simulink model "example8_4"  (R2016b)
settings: Solver=FixedStepDiscrete  StartTime=0.0  StopTime=10.0  RelTol=1e-3  EnableMultiTasking=on
libraries: dspsrcs4 x2, dsparch4 x1, dspadpt3 x1
settings Model: Creator=The MathWorks, Inc.  LastModifiedBy=zhangjin
settings DataIOCC: LimitDataPoints=on  SaveFormat=Array  SignalLoggingName=logsOut
settings OptimizationCC: ExpressionDepthLimit=2147483647  InitFltsAndDblsToZero=on  EfficientMapNaN2IntZero=off  LifeSpan=inf
settings DebuggingCC: SaveWithParameterizedLinksMsg=none  UnderspecifiedInitializationDetection=Classic  MergeDetectMultiDrivingBlocksExec=none  CheckExecutionContextPreStartOutputMsg=on  CheckExecutionContextRuntimeOutputMsg=on  SolverPrmCheckMsg=warning  MultiTaskDSMMsg=warning  MultiTaskCondExecSysMsg=none  FcnCallInpInsideContextMsg=warning  StateNameClashWarn=warning  StrictBusMsg=None  SFUnexpectedBacktrackingDiag=warning  SFNoUnconditionalDefaultTransitionDiag=warning  SFExecutionAtInitializationDiag=none
settings HardwareCC: ProdBitPerPointer=32  ProdBitPerSizeT=32  ProdBitPerPtrDiffT=32  ProdLargestAtomicFloat=None  ProdIntDivRoundTo=Undefined  ProdEndianess=Unspecified  ProdWordSize=32  ProdHWDeviceType=32-bit Generic
settings ModelReferenceCC: UpdateModelReferenceTargets=IfOutOfDate  PropagateSignalLabelsOutOfModel=off
settings GRTTargetCC: TargetFcnLib=ansi_tfl_tmw.mat  TargetLangStandard=C89/C90 (ANSI)  GeneratePreprocessorConditionals=Disable all  CombineOutputUpdateFcns=off  GRTInterface=on
settings ConfigComp: CovMetricSettings=dw  CovHtmlReporting=on  CovSaveCumulativeToWorkspaceVar=on  CovSaveSingleToWorkspaceVar=on  CovExternalEMLEnable=off

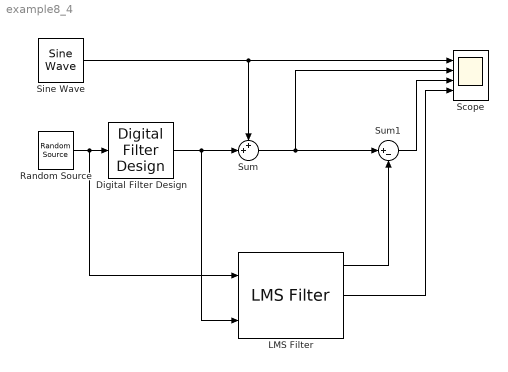
== system example8_4 ==
  Digital Filter Design : dsparch4/Digital Filter Design  mwdsp_browser_bugfix_var=off
  LMS Filter : dspadpt3/LMS Filter  Algo=Normalized LMS  L=32  stepflag=Dialog  mu=0.1  leakage=1.0  ic=0  Adapt=off  resetflag=None  weights=on  secondCoeffMode=User-defined  secondCoeffWordLength=2  secondCoeffFracLength=15  accum2Mode=User-defined  accum2FracLength=20  prodOutput2Mode=User-defined  prodOutput2FracLength=20  prodOutput3Mode=User-defined  prodOutput3FracLength=20  prodOutput4Mode=User-defined  prodOutput4FracLength=20  quotientMode=User-defined  quotientFracLength=20  roundingMode=Floor  overflowMode=off  addnparflag=off
  Random Source : dspsrcs4/Random Source  SrcType=Gaussian  NormMethod=Ziggurat  CltLength=12  MinVal=0  MaxVal=1  MeanVal=0  VarVal=1  RepMode=Specify seed  rawSeed=[23341]  IsInherit=off  SampMode=Discrete  SampTime=0.05  SampFrame=1  DataType=Double  OutComplex=Real  OutputFrames=on
  Scope : Scope  NumInputPorts=4
  Sine Wave : dspsrcs4/Sine Wave  Amplitude=1  Frequency=0.5  Phase=0  SampleMode=Discrete  OutComplex=Real  CompMethod=Trigonometric fcn  TableSize=Speed  SampleTime=0.05  SamplesPerFrame=1  ResetState=Restart at time zero  OutputFrames=on  dataType=double  wordLen=16  udDataType=sfix(16)  fracBitsMode=Best precision  numFracBits=15  OutDataTypeStr=double  LastOutDataTypeStr=double
  Sum : Sum  Inputs=++|
  Sum1 : Sum  Inputs=|+-
  wires:
  Sine Wave/1 -> Scope/1, Sum/1
  Sum/1 -> Sum1/1, Scope/2
  Random Source/1 -> LMS Filter/1, Digital Filter Design/1
  Digital Filter Design/1 -> LMS Filter/2, Sum/2
  LMS Filter/1 -> Sum1/2
  Sum1/1 -> Scope/3
  LMS Filter/2 -> Scope/4
